simulink model "ereg_controller_model"  (R2025b)
settings: Solver=FixedStepDiscrete  StartTime=0.0  StopTime=10.0  RelTol=1e-3
undefined symbols (not defined in the file): Ts_ctrl
settings Model: Creator=ethan  LastModifiedBy=ethan
settings OptimizationCC: DefaultParameterBehavior=Inlined  EnhancedBackFolding=on  PassReuseOutputArgsAs=Individual arguments  ZeroExternalMemoryAtStartup=off  ZeroInternalMemoryAtStartup=off  OptimizeBlockOrder=speed  DifferentSizesBufferReuse=on  OptimizationCustomize=off  EfficientTunableParamExpr=on
settings DebuggingCC: AlgebraicLoopMsg=error  ParameterTunabilityLossMsg=error
settings SFSimCC: MATLABDynamicMemAlloc=off
settings RTWCC: SystemTargetFile=ert.tlc  GenCodeOnly=on  TemplateMakefile=ert_default_tmf  Description=Embedded Coder
settings CodeAppCC: ForceParamTrailComments=on  IgnoreCustomStorageClasses=off  OperatorAnnotations=on  SimulinkDataObjDesc=on  SFDataObjDesc=on  InsertBlockDesc=on
settings ERTTargetCC: ERTCustomFileTemplate=example_file_process.tlc  TargetLangStandard=C99 (ISO)  GenerateSampleERTMain=on

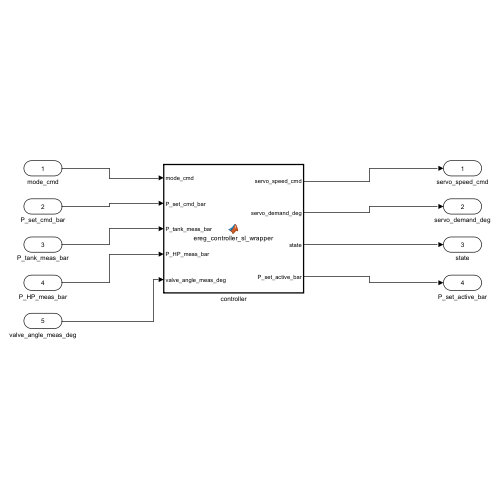
[thumbnail: Simulink's stored preview of the top-level diagram]
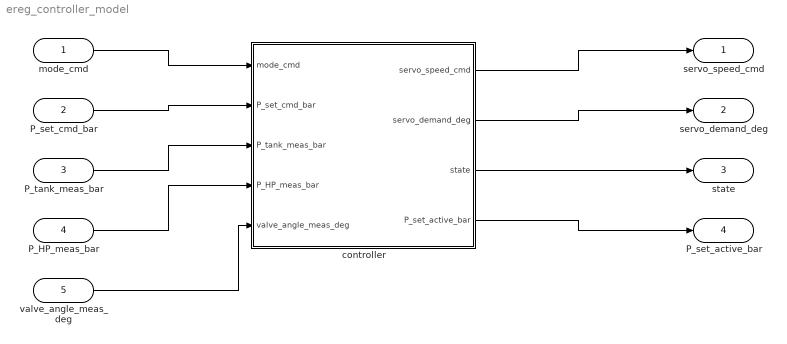
== system ereg_controller_model ==
  mode_cmd : Inport  SampleTime=Ts_ctrl
  P_set_cmd_bar : Inport  Port=2  SampleTime=Ts_ctrl
  P_tank_meas_bar : Inport  Port=3  SampleTime=Ts_ctrl
  P_HP_meas_bar : Inport  Port=4  SampleTime=Ts_ctrl
  valve_angle_meas_deg : Inport  Port=5  SampleTime=Ts_ctrl
  controller : MATLAB Function  TreatAsAtomicUnit=on
  servo_speed_cmd : Outport
  servo_demand_deg : Outport  Port=2
  state : Outport  Port=3
  P_set_active_bar : Outport  Port=4
  wires:
  mode_cmd/1 -> controller/1(mode_cmd)
  P_set_cmd_bar/1 -> controller/2(P_set_cmd_bar)
  P_tank_meas_bar/1 -> controller/3(P_tank_meas_bar)
  P_HP_meas_bar/1 -> controller/4(P_HP_meas_bar)
  valve_angle_meas_deg/1 -> controller/5(valve_angle_meas_deg)
  controller/1(servo_speed_cmd) -> servo_speed_cmd/1
  controller/2(servo_demand_deg) -> servo_demand_deg/1
  controller/3(state) -> state/1
  controller/4(P_set_active_bar) -> P_set_active_bar/1

== matlab function ereg_controller_model/controller ==
  data: mode_cmd input; servo_speed_cmd output; P_set_cmd_bar input; P_tank_meas_bar input; P_HP_meas_bar input; valve_angle_meas_deg input; servo_demand_deg output; state output; P_set_active_bar output; ctrl_params parameter
function [servo_speed_cmd, servo_demand_deg, state, P_set_active_bar] = ...
    ereg_controller_sl_wrapper(mode_cmd, P_set_cmd_bar, P_tank_meas_bar, ...
                               P_HP_meas_bar, valve_angle_meas_deg, ctrl_params)
%EREG_CONTROLLER_SL_WRAPPER Script of the MATLAB Function block in
% ereg_controller_model.slx (injected at build time by build_controller_model).
% ctrl_params is parameter-scope data resolved from the workspace.
%#codegen
persistent x
if isempty(x)
    x = ereg_controller_init();
end
[servo_speed_cmd, servo_demand_deg, state, P_set_active_bar, x] = ereg_controller_step( ...
    mode_cmd, P_set_cmd_bar, P_tank_meas_bar, P_HP_meas_bar, valve_angle_meas_deg, ...
    x, ctrl_params);
end
